simulink model "canonball"  (R2020a)
settings: Solver=VariableStepAuto  StartTime=0.0  StopTime=10.0  RelTol=1e-3
undefined symbols (not defined in the file): drag_coff, theta
libraries: simulink x1
settings Model: Creator=sarbojit  LastModifiedBy=sarbojit

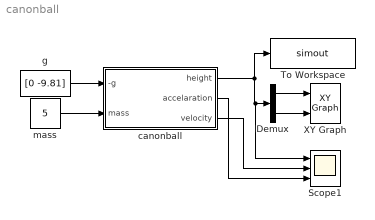
== system canonball ==
  Demux : Demux  Outputs=2
  Scope1 : Scope  NumInputPorts=3
  To Workspace : ToWorkspace  VariableName=simout  SampleTime=-1
  XY Graph : simulink/Sinks/XY Graph  xmin=0  xmax=400  ymin=-10  ymax=200  st=-1
  canonball : Subsystem
  g : Constant  Value=[0 -9.81]
  mass : Constant  Value=5
  wires:
  canonball/1(height) -> To Workspace/1, Scope1/1, Demux/1
  canonball/3(velocity) -> Scope1/2
  mass/1 -> canonball/2(mass)
  Demux/2 -> XY Graph/2
  g/1 -> canonball/1(-g)
  Demux/1 -> XY Graph/1
  canonball/2(accelaration) -> Scope1/3

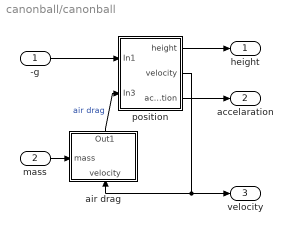
== system canonball/canonball ==
  -g : Inport
  mass : Inport  Port=2
  air drag : Subsystem
      settings: PortSchema="{\"entries\":[{\"content\":{\"sides\":[{\"content\":{\"connectorIds\":[\"In1\"]},\"type\":\"ConnectorPlacement.EquallySpacedRectSide\",\"uuid\":\"eff0201c-5696-466b-9663-78baec171fcf\"},{\"content\":{\"connectorIds\":[\"Out1\"],\"side\":\"RIGHT\"},\"type\":\"ConnectorPlacement.EquallySpacedRectSide\",\"uuid\":\"e5726ea1-319f-48aa-b213-fbd61e592c3c\"},{\"content\":{\"connectorIds\":[\"In2\"],\"side\":\"TOP\"},\"type\":\"ConnectorPlacement.EquallySpacedRectSide\",\"uuid\":\"967e38cb-101e-41a7-8acc-363003834573\"}]},\"type\":\"ConnectorPlacement.EquallySpacedConnector\",\"uuid\":\"439cb318-c5ec-445e-8aa8-2f5e6a6c5f99\"}],\"packageUris\":[\"http://schema.mathworks.com/mf0/Connector/19700101\"],\"version\":\"1.0\"}"
  position : Subsystem
  height : Outport
  accelaration : Outport  Port=2
  velocity : Outport  Port=3
  wires:
  air drag/1(Out1) -> position/2(In3)  "air drag"
  -g/1 -> position/1(In1)
  position/3(accelaration) -> accelaration/1
  mass/1 -> air drag/2(mass)
  position/1(height) -> height/1
  position/2(velocity) -> velocity/1, air drag/1(velocity)

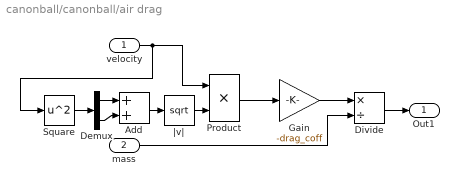
== system canonball/canonball/air drag ==
  velocity : Inport
  mass : Inport  Port=2
  Add : Sum
  Demux : Demux  Outputs=2
  Divide : Product  Inputs=*/
  Gain : Gain  Gain=-drag_coff
  Product : Product
  Square : Math  Operator=square  SaturateOnIntegerOverflow=on
  |v| : Sqrt  SaturateOnIntegerOverflow=on
  Out1 : Outport
  wires:
  mass/1 -> Divide/2
  Gain/1 -> Divide/1
  Product/1 -> Gain/1
  velocity/1 -> Square/1, Product/1
  Divide/1 -> Out1/1
  Square/1 -> Demux/1
  Demux/1 -> Add/1
  Demux/2 -> Add/2
  Add/1 -> |v|/1
  |v|/1 -> Product/2

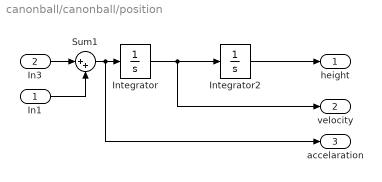
== system canonball/canonball/position ==
  In1 : Inport
  In3 : Inport  Port=2
  Integrator : Integrator  InitialCondition=100*[cosd(theta) sind(theta)]
  Integrator2 : Integrator  InitialCondition=[0 0]  LimitOutput=on  UpperSaturationLimit=[inf inf]  LowerSaturationLimit=[0 0]
  Sum1 : Sum  Inputs=|++
  height : Outport
  velocity : Outport  Port=2
  accelaration : Outport  Port=3
  wires:
  Integrator/1 -> velocity/1, Integrator2/1
  In1/1 -> Sum1/2
  In3/1 -> Sum1/1
  Sum1/1 -> accelaration/1, Integrator/1
  Integrator2/1 -> height/1
